simulink model "LT_TM200"  (R2025b)
settings: Solver=FixedStepAuto  StartTime=0.0  StopTime=inf  FixedStep=1E-3  RelTol=1e-3
settings Model: Creator=abstract  LastModifiedBy=abstract

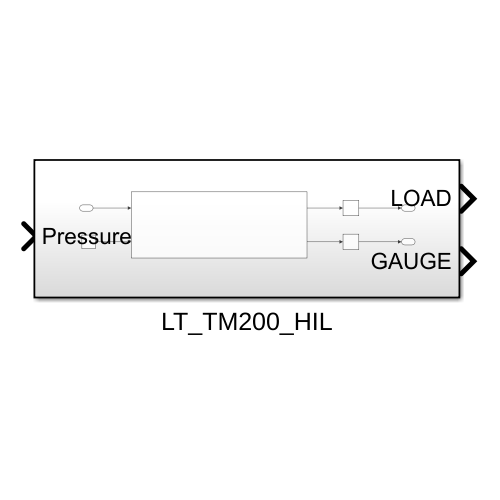
[thumbnail: Simulink's stored preview of the top-level diagram]
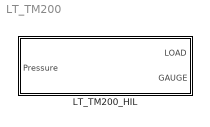
== system LT_TM200 ==
  LT_TM200_HIL : Subsystem

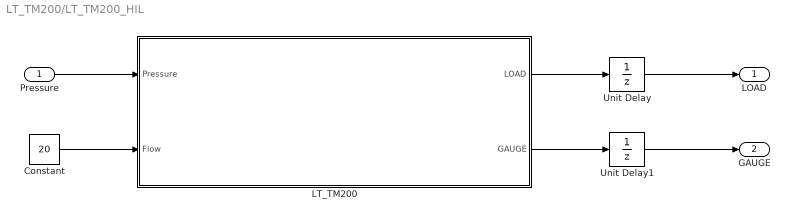
== system LT_TM200/LT_TM200_HIL ==
  Pressure : Inport  OutDataTypeStr=single
  Constant : Constant  Value=20  OutDataTypeStr=Inherit: Inherit via back propagation  SampleTime=-1
  LT_TM200 : MATLAB Function  TreatAsAtomicUnit=on
  Unit Delay : UnitDelay  SampleTime=-1  HasFrameUpgradeWarning=on
  Unit Delay1 : UnitDelay  SampleTime=-1  HasFrameUpgradeWarning=on
  LOAD : Outport  OutDataTypeStr=single
  GAUGE : Outport  Port=2  OutDataTypeStr=int16
  wires:
  Unit Delay1/1 -> GAUGE/1
  LT_TM200/2(GAUGE) -> Unit Delay1/1
  Pressure/1 -> LT_TM200/1(Pressure)
  Constant/1 -> LT_TM200/2(Flow)
  Unit Delay/1 -> LOAD/1
  LT_TM200/1(LOAD) -> Unit Delay/1

== matlab function LT_TM200/LT_TM200_HIL/LT_TM200 ==
  data: Pressure input; Flow input; LOAD output; GAUGE output
function [LOAD, GAUGE] = LT_TM200(Pressure, Flow)

Set_TM_Pressure(Pressure);
Set_TM_FLow(Flow);

[LOAD, GAUGE] = Get_TM_State();
